simulink model "PLL"  (R2013a)
settings: Solver=ode45  StartTime=0.0  StopTime=1200/1200  FixedStep=1e-6  RelTol=1/(1200*2048)
values from neighbouring files (symbols this model uses):
  Gain = 1 * 10^4    (= 10000)    [PLL.m]
  K = (16*1200*sqrt(1200)/0.707)^2    [PLL.m]
  wcut = fcut*2*pi    (= 7539.82236862)    [PLL.m]
  wn = r(1)    [PLL.m]
libraries: commsynccomp2 x2, dsparch4 x1
settings Model: Creator=Cedric  LastModifiedBy=Cedric

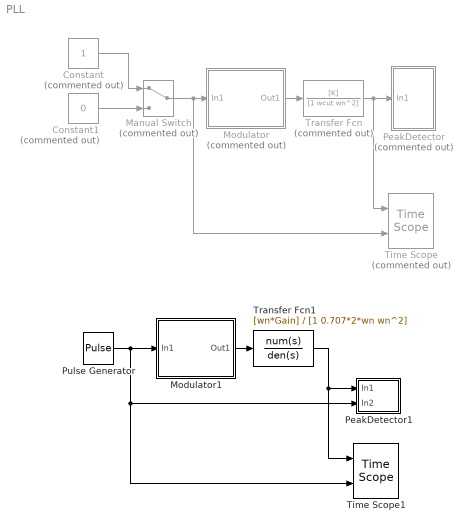
== system PLL ==
  Constant : Constant  Commented=on
  Constant1 : Constant  Commented=on  Value=0
  Manual Switch : ManualSwitch  Commented=on
  Modulator : Subsystem  Commented=on
  Modulator1 : Subsystem
  PeakDetector : Subsystem  Commented=on
  PeakDetector1 : Subsystem
  Pulse Generator : DiscretePulseGenerator  PulseType=Time based  Period=1/(600)  PulseWidth=50
  Time Scope : TimeScope  Commented=on  NumInputPorts=2  DefaultConfigurationName=spbscopes.TimeScopeBlockCfg
      settings: CopyFcn=scopeextensions.ScopeBlock.callback(gcbh, 'onBlockCopy', gcbh);  DeleteFcn=scopeextensions.ScopeBlock.callback(gcbh, 'onBlockDelete');  PreSaveFcn=scopeextensions.ScopeBlock.callback(gcbh, 'onModelSave');  NameChangeFcn=scopeextensions.ScopeBlock.callback(gcbh, 'onBlockRename');  CloseFcn=scopeextensions.ScopeBlock.callback(gcbh, 'onBlockClose');  PreDeleteFcn=scopeextensions.ScopeBlock.callback(gcbh, 'onBlockPreDelete');
  Time Scope1 : TimeScope  NumInputPorts=2  DefaultConfigurationName=spbscopes.TimeScopeBlockCfg
      settings: CopyFcn=scopeextensions.ScopeBlock.callback(gcbh, 'onBlockCopy', gcbh);  DeleteFcn=scopeextensions.ScopeBlock.callback(gcbh, 'onBlockDelete');  PreSaveFcn=scopeextensions.ScopeBlock.callback(gcbh, 'onModelSave');  NameChangeFcn=scopeextensions.ScopeBlock.callback(gcbh, 'onBlockRename');  CloseFcn=scopeextensions.ScopeBlock.callback(gcbh, 'onBlockClose');  PreDeleteFcn=scopeextensions.ScopeBlock.callback(gcbh, 'onBlockPreDelete');
  Transfer Fcn : TransferFcn  Commented=on  Numerator=[K]  Denominator=[1 wcut wn^2]
  Transfer Fcn1 : TransferFcn  Numerator=[wn*Gain]  Denominator=[1 0.707*2*wn wn^2]
  wires:
  Constant/1 -> Manual Switch/1
  Constant1/1 -> Manual Switch/2
  Modulator/1(Out1) -> Transfer Fcn/1
  Transfer Fcn/1 -> Time Scope/1, PeakDetector/1(In1)
  Manual Switch/1 -> Time Scope/2, Modulator/1(In1)
  Modulator1/1(Out1) -> Transfer Fcn1/1
  Transfer Fcn1/1 -> Time Scope1/1, PeakDetector1/1(In1)
  Pulse Generator/1 -> Time Scope1/2, PeakDetector1/2(In2), Modulator1/1(In1)

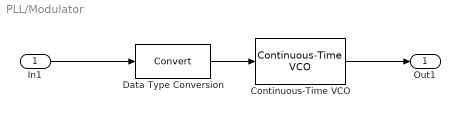
== system PLL/Modulator ==
  In1 : Inport
  Continuous-Time VCO : commsynccomp2/Continuous-Time VCO  Ac=1  Fc=1200  Kc=1000  Ph=0
  Data Type Conversion : DataTypeConversion
  Out1 : Outport
  wires:
  In1/1 -> Data Type Conversion/1
  Data Type Conversion/1 -> Continuous-Time VCO/1
  Continuous-Time VCO/1 -> Out1/1

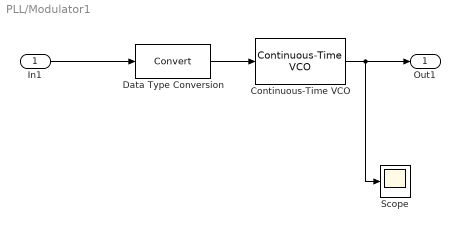
== system PLL/Modulator1 ==
  In1 : Inport
  Continuous-Time VCO : commsynccomp2/Continuous-Time VCO  Ac=1  Fc=1200  Kc=1000  Ph=0
  Data Type Conversion : DataTypeConversion
  Scope : Scope
      settings: TimeRange=0.007754789272030654  YMin=0.06833333333333358  YMax=0.101666666666667  SaveName=ScopeData4
  Out1 : Outport
  wires:
  In1/1 -> Data Type Conversion/1
  Data Type Conversion/1 -> Continuous-Time VCO/1
  Continuous-Time VCO/1 -> Scope/1, Out1/1

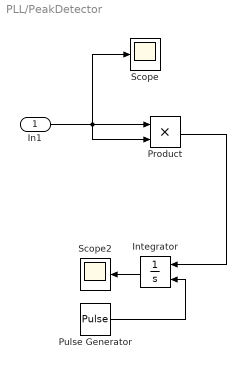
== system PLL/PeakDetector ==
  In1 : Inport
  Integrator : Integrator  ExternalReset=rising
  Product : Product
  Pulse Generator : DiscretePulseGenerator  Period=256  PulseWidth=128  SampleTime=1/(1200*256)
  Scope : Scope
      settings: YMin=-0.45  YMax=0.45
  Scope2 : Scope
      settings: SaveName=ScopeData2
  wires:
  In1/1 -> Product/2, Product/1, Scope/1
  Pulse Generator/1 -> Integrator/2
  Product/1 -> Integrator/1
  Integrator/1 -> Scope2/1

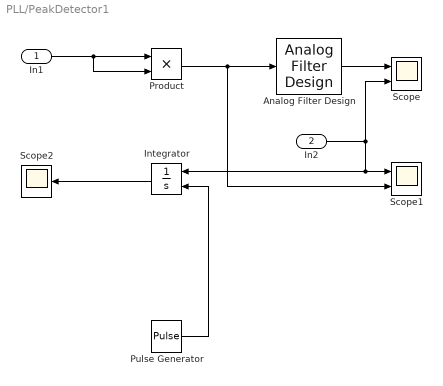
== system PLL/PeakDetector1 ==
  In1 : Inport
  In2 : Inport  Port=2
  Analog Filter Design : dsparch4/Analog Filter Design  method=Butterworth  filttype=Lowpass  N=2  Wlo=2*pi*1000  Whi=80  Rp=2  Rs=40
  Integrator : Integrator  ExternalReset=rising
  Product : Product
  Pulse Generator : DiscretePulseGenerator  Period=256  PulseWidth=128  SampleTime=1/(1200*256)
  Scope : Scope  NumInputPorts=2
      settings: YMin=-1.73472e-17~-5  YMax=0.24~5
  Scope1 : Scope  NumInputPorts=2
      settings: YMin=-1.73472e-17~-5  YMax=0.24~5  SaveName=ScopeData3
  Scope2 : Scope
      settings: SaveName=ScopeData2
  wires:
  In1/1 -> Product/2, Product/1
  Pulse Generator/1 -> Integrator/2
  Integrator/1 -> Scope2/1
  Product/1 -> Analog Filter Design/1, Scope1/2
  In2/1 -> Integrator/1, Scope1/1, Scope/2
  Analog Filter Design/1 -> Scope/1
